simulink model "SigmaDelta"  (R2021b)
settings: Solver=VariableStepAuto  StartTime=0.0  StopTime=1  RelTol=1e-3
PreLoadFcn:
  | load DecFir.mat
undefined symbols (not defined in the file or in its folder): designMultirateFIR
libraries: dspmlti4 x6
settings Model: Creator=Utente  LastModifiedBy=Utente

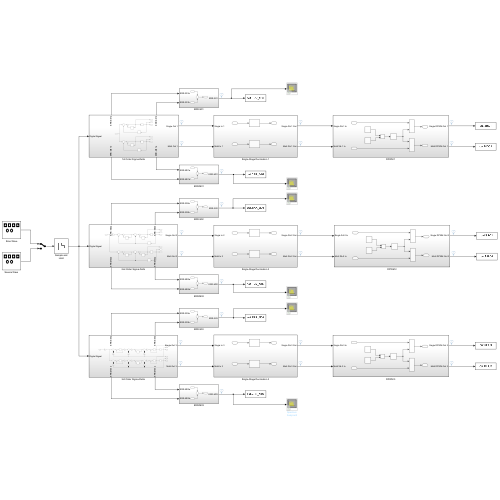
[thumbnail: Simulink's stored preview of the top-level diagram]
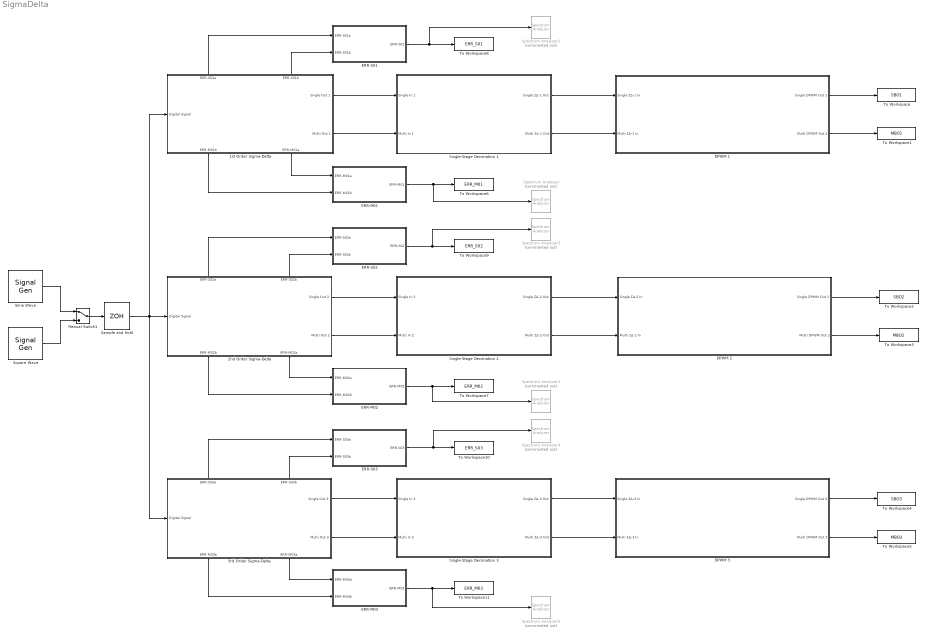
== system SigmaDelta ==
  "1st Order Sigma-Delta " : Subsystem
      settings: PortSchema="{\"entries\":[{\"content\":{\"sides\":[{\"content\":{\"connectorIds\":[\"In1\"]},\"type\":\"ConnectorPlacement.EquallySpacedRectSide\",\"uuid\":\"386a8987-fa85-4bfc-abbe-97ad6325c10a\"},{\"content\":{\"connectorIds\":[\"Out1\",\"Out2\"],\"side\":\"RIGHT\"},\"type\":\"ConnectorPlacement.EquallySpacedRectSide\",\"uuid\":\"605e7def-dc36-4f80-8847-9394a6da716c\"},{\"content\":{\"connectorIds\":[\"Out5\",\"Out6\"],\"side\":\"TOP\"},\"type\":\"ConnectorPlacement.EquallySpacedRectSide\",\"uuid\":\"bb7b67fd-46b8-47e1-a371-5b31483f4377\"},{\"content\":{\"connectorIds\":[\"Out3\",\"Out4\"],\"side\":\"BOTTOM\"},\"type\":\"ConnectorPlacement.EquallySpacedRectSide\",\"uuid\":\"407ca7d6-6743-42b4-90a6-330882115c21\"}]},\"type\":\"ConnectorPlacement.EquallySpacedConnector\",\"uuid\":\"38d6658d-cd74-4f08-86e0-cb3a607ff030\"}],\"packageUris\":[\"http://schema.mathworks.com/mf0/Connector/R2020b\"],\"version\":\"1.0\"}"
  2nd Order Sigma-Delta : Subsystem
      settings: PortSchema="{\"entries\":[{\"content\":{\"sides\":[{\"content\":{\"connectorIds\":[\"In1\"]},\"type\":\"ConnectorPlacement.EquallySpacedRectSide\",\"uuid\":\"386a8987-fa85-4bfc-abbe-97ad6325c10a\"},{\"content\":{\"connectorIds\":[\"Out1\",\"Out2\"],\"side\":\"RIGHT\"},\"type\":\"ConnectorPlacement.EquallySpacedRectSide\",\"uuid\":\"605e7def-dc36-4f80-8847-9394a6da716c\"},{\"content\":{\"connectorIds\":[\"Out5\",\"Out6\"],\"side\":\"TOP\"},\"type\":\"ConnectorPlacement.EquallySpacedRectSide\",\"uuid\":\"bb7b67fd-46b8-47e1-a371-5b31483f4377\"},{\"content\":{\"connectorIds\":[\"Out3\",\"Out4\"],\"side\":\"BOTTOM\"},\"type\":\"ConnectorPlacement.EquallySpacedRectSide\",\"uuid\":\"9f9d581d-12dd-4703-9574-97e4d852a146\"}]},\"type\":\"ConnectorPlacement.EquallySpacedConnector\",\"uuid\":\"38d6658d-cd74-4f08-86e0-cb3a607ff030\"}],\"packageUris\":[\"http://schema.mathworks.com/mf0/Connector/R2020b\"],\"version\":\"1.0\"}"
  3rd Order Sigma-Delta : Subsystem
      settings: PortSchema="{\"entries\":[{\"content\":{\"sides\":[{\"content\":{\"connectorIds\":[\"In1\"]},\"type\":\"ConnectorPlacement.EquallySpacedRectSide\",\"uuid\":\"358bd809-644a-47c9-aee6-c26862502fbd\"},{\"content\":{\"connectorIds\":[\"Out1\",\"Out2\"],\"side\":\"RIGHT\"},\"type\":\"ConnectorPlacement.EquallySpacedRectSide\",\"uuid\":\"63769fbe-dbed-44df-abee-7514b671db90\"},{\"content\":{\"connectorIds\":[\"Out5\",\"Out6\"],\"side\":\"TOP\"},\"type\":\"ConnectorPlacement.EquallySpacedRectSide\",\"uuid\":\"5696ef81-7309-4688-a911-424d4e0695b6\"},{\"content\":{\"connectorIds\":[\"Out3\",\"Out4\"],\"side\":\"BOTTOM\"},\"type\":\"ConnectorPlacement.EquallySpacedRectSide\",\"uuid\":\"575d4fed-9583-4a67-98b3-10e8b887a15e\"}]},\"type\":\"ConnectorPlacement.EquallySpacedConnector\",\"uuid\":\"3f568709-b940-42e7-9c29-4ecbd340a24d\"}],\"packageUris\":[\"http://schema.mathworks.com/mf0/Connector/R2020b\"],\"version\":\"1.0\"}"
  DPWM 1 : Subsystem
  DPWM 2 : Subsystem
  DPWM 3 : Subsystem
  ERR-M01 : Subsystem
  ERR-M02 : Subsystem
  ERR-M03 : Subsystem
  ERR-S01 : Subsystem
  ERR-S02 : Subsystem
  ERR-S03 : Subsystem
  Manual Switch1 : ManualSwitch
  Sample and Hold : ZeroOrderHold  SampleTime=1/(48e3*64)
  Siine Wave : SignalGenerator  Frequency=6283  Units=rad/sec
  Single-Stage Decimation 1 : Subsystem
  Single-Stage Decimation 2 : Subsystem
  Single-Stage Decimation 3 : Subsystem
  Spectrum Analyzer{,1..5} (6 alike) : SpectrumAnalyzer  Commented=on
  Square Wave : SignalGenerator  WaveForm=square  Frequency=6283  Units=rad/sec
  To Workspace : ToWorkspace  VariableName=SBO1  SaveFormat=Timeseries  SampleTime=-1
  To Workspace1 : ToWorkspace  VariableName=MBO1  SaveFormat=Timeseries  SampleTime=-1
  To Workspace10 : ToWorkspace  VariableName=ERR_S03  SaveFormat=Timeseries  SampleTime=-1
  To Workspace11 : ToWorkspace  VariableName=ERR_M03  SaveFormat=Timeseries  SampleTime=-1
  To Workspace2 : ToWorkspace  VariableName=SBO2  SaveFormat=Timeseries  SampleTime=-1
  To Workspace3 : ToWorkspace  VariableName=MBO2  SaveFormat=Timeseries  SampleTime=-1
  To Workspace4 : ToWorkspace  VariableName=SBO3  SaveFormat=Timeseries  SampleTime=-1
  To Workspace5 : ToWorkspace  VariableName=MBO3  SaveFormat=Timeseries  SampleTime=-1
  To Workspace6 : ToWorkspace  VariableName=ERR_M01  SaveFormat=Timeseries  SampleTime=-1
  To Workspace7 : ToWorkspace  VariableName=ERR_M02  SaveFormat=Timeseries  SampleTime=-1
  To Workspace8 : ToWorkspace  VariableName=ERR_S01  SaveFormat=Timeseries  SampleTime=-1
  To Workspace9 : ToWorkspace  VariableName=ERR_S02  SaveFormat=Timeseries  SampleTime=-1
  wires:
  Square Wave/1 -> Manual Switch1/2
  DPWM 1/2(Multi DPWM Out 1) -> To Workspace1/1
  DPWM 1/1(Single DPWM Out 1) -> To Workspace/1
  3rd Order Sigma-Delta/2(Multi Out 3) -> Single-Stage Decimation 3/2(Multi In 3)
  3rd Order Sigma-Delta/1(Single Out 3) -> Single-Stage Decimation 3/1(Single In 3)
  Single-Stage Decimation 3/2(Multi ΣΔ-3 Out) -> DPWM 3/2(Multi ΣΔ-3 In)
  Single-Stage Decimation 3/1(Single ΣΔ-3 Out) -> DPWM 3/1(Single ΣΔ-3 In)
  DPWM 3/1(Single DPWM Out 3) -> To Workspace4/1
  Single-Stage Decimation 1/1(Single ΣΔ-1 Out) -> DPWM 1/1(Single ΣΔ-1 In)
  "1st Order Sigma-Delta "/2(" Multi Out 1") -> Single-Stage Decimation 1/2(Multi In 1)
  "1st Order Sigma-Delta "/1(Single Out 1) -> Single-Stage Decimation 1/1(Single In 1)
  DPWM 2/2(Multi DPWM Out 2) -> To Workspace3/1
  Manual Switch1/1 -> Sample and Hold/1
  DPWM 2/1(Single DPWM Out 2) -> To Workspace2/1
  Single-Stage Decimation 1/2(Multi ΣΔ-1 Out) -> DPWM 1/2(Multi ΣΔ-1 In)
  2nd Order Sigma-Delta/1(Single Out 2) -> Single-Stage Decimation 2/1(Single In 2)
  DPWM 3/2(Multi DPWM Out 3) -> To Workspace5/1
  Sample and Hold/1 -> "1st Order Sigma-Delta "/1(Digital Signal), 3rd Order Sigma-Delta/1(Digital Signal), 2nd Order Sigma-Delta/1(Digital Signal)
  Siine Wave/1 -> Manual Switch1/1
  Single-Stage Decimation 2/2(Multi ΣΔ-2 Out) -> DPWM 2/2(Multi ΣΔ-2 In)
  Single-Stage Decimation 2/1(Single ΣΔ-2 Out) -> DPWM 2/1(Single ΣΔ-2 In)
  2nd Order Sigma-Delta/2(" Multi Out 2") -> Single-Stage Decimation 2/2(Multi In 2)
  ERR-M01/1(ERR-M01) -> Spectrum Analyzer/1, To Workspace6/1
  "1st Order Sigma-Delta "/4(ERR-M01a) -> ERR-M01/1(ERR-M01a)
  "1st Order Sigma-Delta "/3(ERR-M01b) -> ERR-M01/2(ERR-M01b)
  2nd Order Sigma-Delta/4(ERR-M02a) -> ERR-M02/1(ERR-M02a)
  2nd Order Sigma-Delta/3(ERR-M02b) -> ERR-M02/2(ERR-M02b)
  ERR-S01/1(ERR-S01) -> Spectrum Analyzer2/1, To Workspace8/1
  "1st Order Sigma-Delta "/6(ERR-S01b) -> ERR-S01/2(ERR-S01b)
  "1st Order Sigma-Delta "/5(ERR-S01a) -> ERR-S01/1(ERR-S01a)
  ERR-S02/1(ERR-S02) -> Spectrum Analyzer3/1, To Workspace9/1
  2nd Order Sigma-Delta/5(ERR-S02a) -> ERR-S02/1(ERR-S02a)
  2nd Order Sigma-Delta/6(ERR-S02b) -> ERR-S02/2(ERR-S02b)
  ERR-M02/1(ERR-M02) -> Spectrum Analyzer1/1, To Workspace7/1
  3rd Order Sigma-Delta/6(ERR-S03b) -> ERR-S03/2(ERR-S03b)
  ERR-S03/1(ERR-S03) -> Spectrum Analyzer4/1, To Workspace10/1
  3rd Order Sigma-Delta/5(ERR-S03a) -> ERR-S03/1(ERR-S03a)
  3rd Order Sigma-Delta/3(ERR-M03b) -> ERR-M03/2(ERR-M03b)
  ERR-M03/1(ERR-M03) -> Spectrum Analyzer5/1, To Workspace11/1
  3rd Order Sigma-Delta/4(ERR-M03a) -> ERR-M03/1(ERR-M03a)

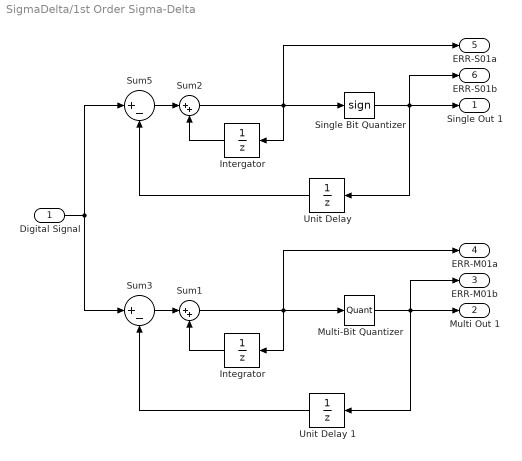
== system SigmaDelta/1st Order Sigma-Delta  ==
  Digital Signal : Inport
  Integrator : UnitDelay  SampleTime=-1  HasFrameUpgradeWarning=on
  Intergator : UnitDelay  SampleTime=-1  HasFrameUpgradeWarning=on
  Multi-Bit Quantizer : Quantizer  QuantizationInterval=0.15
  Single Bit Quantizer : Signum
  Sum1 : Sum  Inputs=|++
  Sum2 : Sum  Inputs=|++
  Sum3 : Sum  Inputs=|+-  AccumDataTypeStr=double  SampleTime=1/(48e3*64)
  Sum5 : Sum  Inputs=|+-  AccumDataTypeStr=double  SampleTime=1/(48e3*64)
  Unit Delay : UnitDelay  SampleTime=-1  HasFrameUpgradeWarning=on
  Unit Delay 1 : UnitDelay  SampleTime=-1  HasFrameUpgradeWarning=on
  Single Out 1 : Outport
  " Multi Out 1" : Outport  Port=2  OutDataTypeStr=double
  ERR-M01b : Outport  Port=3  OutDataTypeStr=double
  ERR-M01a : Outport  Port=4  OutDataTypeStr=double
  ERR-S01a : Outport  Port=5  OutDataTypeStr=double
  ERR-S01b : Outport  Port=6  OutDataTypeStr=double
  wires:
  Unit Delay/1 -> Sum5/2
  Intergator/1 -> Sum2/2
  Sum5/1 -> Sum2/1
  Unit Delay 1/1 -> Sum3/2
  Integrator/1 -> Sum1/2
  Digital Signal/1 -> Sum5/1, Sum3/1
  Sum3/1 -> Sum1/1
  Sum1/1 -> ERR-M01a/1, Multi-Bit Quantizer/1, Integrator/1
  Multi-Bit Quantizer/1 -> " Multi Out 1"/1, Unit Delay 1/1, ERR-M01b/1
  Sum2/1 -> ERR-S01a/1, Intergator/1, Single Bit Quantizer/1
  Single Bit Quantizer/1 -> ERR-S01b/1, Unit Delay/1, Single Out 1/1

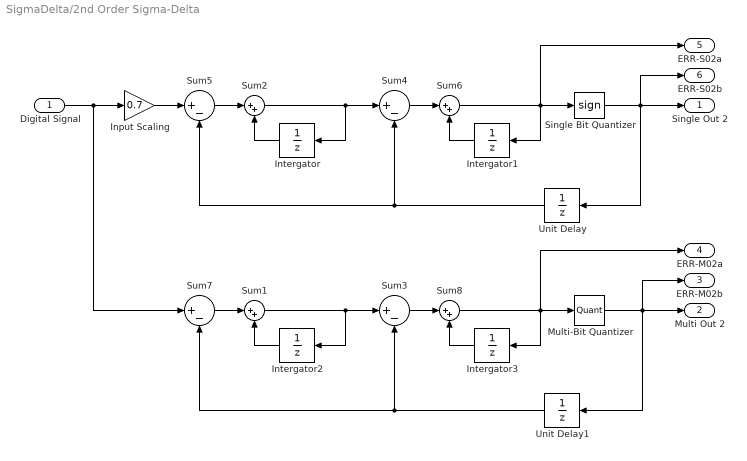
== system SigmaDelta/2nd Order Sigma-Delta ==
  Digital Signal : Inport
  Input Scaling : Gain  Gain=0.7  SampleTime=1/(48e3*64)
  Intergator{,1..3} (4 alike) : UnitDelay  SampleTime=-1  HasFrameUpgradeWarning=on
  Multi-Bit Quantizer : Quantizer  QuantizationInterval=0.15
  Single Bit Quantizer : Signum
  Sum{1..2,6,8} (4 alike) : Sum  Inputs=|++
  Sum{3..5,7} (4 alike) : Sum  Inputs=|+-  AccumDataTypeStr=double  SampleTime=1/(48e3*64)
  Unit Delay : UnitDelay  SampleTime=-1  HasFrameUpgradeWarning=on
  Unit Delay1 : UnitDelay  SampleTime=-1  HasFrameUpgradeWarning=on
  Single Out 2 : Outport
  " Multi Out 2" : Outport  Port=2  OutDataTypeStr=double
  ERR-M02b : Outport  Port=3  OutDataTypeStr=double
  ERR-M02a : Outport  Port=4  OutDataTypeStr=double
  ERR-S02a : Outport  Port=5  OutDataTypeStr=double
  ERR-S02b : Outport  Port=6  OutDataTypeStr=double
  wires:
  Sum2/1 -> Sum4/1, Intergator/1
  Unit Delay/1 -> Sum4/2, Sum5/2
  Intergator/1 -> Sum2/2
  Sum5/1 -> Sum2/1
  Input Scaling/1 -> Sum5/1
  Sum4/1 -> Sum6/1
  Intergator1/1 -> Sum6/2
  Sum3/1 -> Sum8/1
  Sum7/1 -> Sum1/1
  Intergator2/1 -> Sum1/2
  Sum1/1 -> Sum3/1, Intergator2/1
  Unit Delay1/1 -> Sum3/2, Sum7/2
  Digital Signal/1 -> Sum7/1, Input Scaling/1
  Intergator3/1 -> Sum8/2
  Sum8/1 -> ERR-M02a/1, Multi-Bit Quantizer/1, Intergator3/1
  Multi-Bit Quantizer/1 -> Unit Delay1/1, " Multi Out 2"/1, ERR-M02b/1
  Sum6/1 -> ERR-S02a/1, Single Bit Quantizer/1, Intergator1/1
  Single Bit Quantizer/1 -> Unit Delay/1, ERR-S02b/1, Single Out 2/1

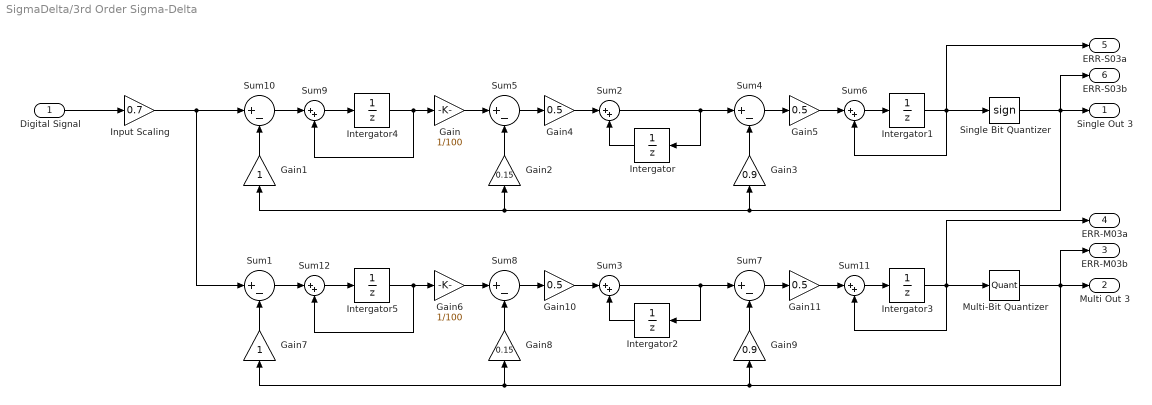
== system SigmaDelta/3rd Order Sigma-Delta ==
  Digital Signal : Inport
  Gain : Gain  Gain=1/100
  Gain1 : Gain
  Gain{4..5,10..11} (4 alike) : Gain  Gain=0.5
  Gain2 : Gain  Gain=0.15
  Gain3 : Gain  Gain=0.9
  Gain6 : Gain  Gain=1/100
  Gain7 : Gain
  Gain8 : Gain  Gain=0.15
  Gain9 : Gain  Gain=0.9
  Input Scaling : Gain  Gain=0.7  SampleTime=1/(48e3*64)
  Intergator{,1..5} (6 alike) : UnitDelay  SampleTime=-1  HasFrameUpgradeWarning=on
  Multi-Bit Quantizer : Quantizer  QuantizationInterval=0.15
  Single Bit Quantizer : Signum
  Sum{1,4..5,7..8,10} (6 alike) : Sum  Inputs=|+-  AccumDataTypeStr=double  SampleTime=1/(48e3*64)
  Sum{2..3,6,9,11..12} (6 alike) : Sum  Inputs=|++
  Single Out 3 : Outport
  Multi Out 3 : Outport  Port=2
  ERR-M03b : Outport  Port=3  OutDataTypeStr=double
  ERR-M03a : Outport  Port=4  OutDataTypeStr=double
  ERR-S03a : Outport  Port=5  OutDataTypeStr=double
  ERR-S03b : Outport  Port=6  OutDataTypeStr=double
  wires:
  Sum2/1 -> Sum4/1, Intergator/1
  Intergator/1 -> Sum2/2
  Sum5/1 -> Gain4/1
  Sum6/1 -> Intergator1/1
  Digital Signal/1 -> Input Scaling/1
  Sum10/1 -> Sum9/1
  Sum9/1 -> Intergator4/1
  Intergator4/1 -> Gain/1, Sum9/2
  Gain/1 -> Sum5/1
  Gain1/1 -> Sum10/2
  Gain2/1 -> Sum5/2
  Gain3/1 -> Sum4/2
  Gain4/1 -> Sum2/1
  Sum4/1 -> Gain5/1
  Gain5/1 -> Sum6/1
  Gain7/1 -> Sum1/2
  Intergator5/1 -> Gain6/1, Sum12/2
  Sum12/1 -> Intergator5/1
  Sum1/1 -> Sum12/1
  Gain9/1 -> Sum7/2
  Sum7/1 -> Gain11/1
  Sum11/1 -> Intergator3/1
  Gain10/1 -> Sum3/1
  Sum8/1 -> Gain10/1
  Intergator2/1 -> Sum3/2
  Gain6/1 -> Sum8/1
  Input Scaling/1 -> Sum1/1, Sum10/1
  Gain11/1 -> Sum11/1
  Gain8/1 -> Sum8/2
  Sum3/1 -> Sum7/1, Intergator2/1
  Intergator3/1 -> ERR-M03a/1, Multi-Bit Quantizer/1, Sum11/2
  Multi-Bit Quantizer/1 -> ERR-M03b/1, Gain9/1, Gain7/1, Gain8/1, Multi Out 3/1
  Single Bit Quantizer/1 -> ERR-S03b/1, Gain3/1, Gain1/1, Gain2/1, Single Out 3/1
  Intergator1/1 -> ERR-S03a/1, Single Bit Quantizer/1, Sum6/2

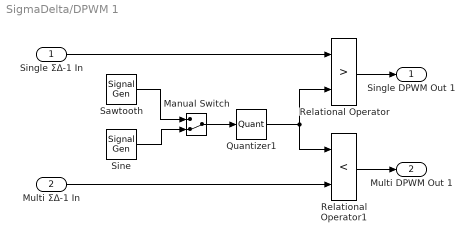
== system SigmaDelta/DPWM 1 ==
  Single ΣΔ-1 In : Inport
  Multi ΣΔ-1 In : Inport  Port=2
  Manual Switch : ManualSwitch  CurrentSetting=0
  Quantizer1 : Quantizer  QuantizationInterval=0.15
  Relational Operator : RelationalOperator  Operator=>  OutDataTypeStr=boolean  RndMeth=Simplest
  Relational Operator1 : RelationalOperator  Operator=<  OutDataTypeStr=boolean  RndMeth=Simplest
  Sawtooth : SignalGenerator  WaveForm=sawtooth  Frequency=1000  Units=rad/sec
  "Sine " : SignalGenerator  Frequency=1000  Units=rad/sec
  Single DPWM Out 1 : Outport
  Multi DPWM Out 1 : Outport  Port=2
  wires:
  Sawtooth/1 -> Manual Switch/1
  "Sine "/1 -> Manual Switch/2
  Manual Switch/1 -> Quantizer1/1
  Single ΣΔ-1 In/1 -> Relational Operator/1
  Quantizer1/1 -> Relational Operator/2, Relational Operator1/1
  Relational Operator/1 -> Single DPWM Out 1/1
  Relational Operator1/1 -> Multi DPWM Out 1/1
  Multi ΣΔ-1 In/1 -> Relational Operator1/2

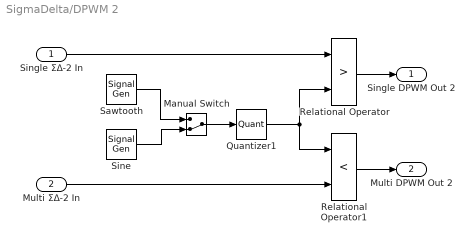
== system SigmaDelta/DPWM 2 ==
  Single ΣΔ-2 In : Inport
  Multi ΣΔ-2 In : Inport  Port=2
  Manual Switch : ManualSwitch  CurrentSetting=0
  Quantizer1 : Quantizer  QuantizationInterval=0.15
  Relational Operator : RelationalOperator  Operator=>  OutDataTypeStr=boolean  RndMeth=Simplest
  Relational Operator1 : RelationalOperator  Operator=<  OutDataTypeStr=boolean  RndMeth=Simplest
  Sawtooth : SignalGenerator  WaveForm=sawtooth  Frequency=1000  Units=rad/sec
  "Sine " : SignalGenerator  Frequency=1000  Units=rad/sec
  Single DPWM Out 2 : Outport
  Multi DPWM Out 2 : Outport  Port=2
  wires:
  Sawtooth/1 -> Manual Switch/1
  "Sine "/1 -> Manual Switch/2
  Manual Switch/1 -> Quantizer1/1
  Single ΣΔ-2 In/1 -> Relational Operator/1
  Quantizer1/1 -> Relational Operator/2, Relational Operator1/1
  Relational Operator/1 -> Single DPWM Out 2/1
  Relational Operator1/1 -> Multi DPWM Out 2/1
  Multi ΣΔ-2 In/1 -> Relational Operator1/2

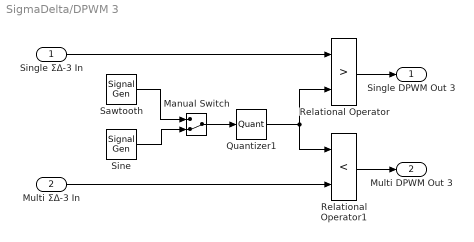
== system SigmaDelta/DPWM 3 ==
  Single ΣΔ-3 In : Inport
  Multi ΣΔ-3 In : Inport  Port=2
  Manual Switch : ManualSwitch  CurrentSetting=0
  Quantizer1 : Quantizer  QuantizationInterval=0.15
  Relational Operator : RelationalOperator  Operator=>  OutDataTypeStr=boolean  RndMeth=Simplest
  Relational Operator1 : RelationalOperator  Operator=<  OutDataTypeStr=boolean  RndMeth=Simplest
  Sawtooth : SignalGenerator  WaveForm=sawtooth  Frequency=1000  Units=rad/sec
  "Sine " : SignalGenerator  Frequency=1000  Units=rad/sec
  Single DPWM Out 3 : Outport
  Multi DPWM Out 3 : Outport  Port=2
  wires:
  Sawtooth/1 -> Manual Switch/1
  "Sine "/1 -> Manual Switch/2
  Manual Switch/1 -> Quantizer1/1
  Single ΣΔ-3 In/1 -> Relational Operator/1
  Quantizer1/1 -> Relational Operator/2, Relational Operator1/1
  Relational Operator/1 -> Single DPWM Out 3/1
  Relational Operator1/1 -> Multi DPWM Out 3/1
  Multi ΣΔ-3 In/1 -> Relational Operator1/2

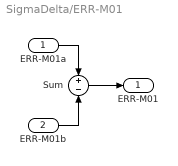
== system SigmaDelta/ERR-M01 ==
  ERR-M01a : Inport
  ERR-M01b : Inport  Port=2
  Sum : Sum  Inputs=+|-
  ERR-M01 : Outport
  wires:
  ERR-M01a/1 -> Sum/1
  ERR-M01b/1 -> Sum/2
  Sum/1 -> ERR-M01/1

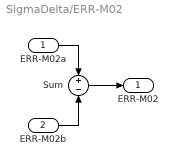
== system SigmaDelta/ERR-M02 ==
  ERR-M02a : Inport
  ERR-M02b : Inport  Port=2
  Sum : Sum  Inputs=+|-
  ERR-M02 : Outport
  wires:
  ERR-M02a/1 -> Sum/1
  ERR-M02b/1 -> Sum/2
  Sum/1 -> ERR-M02/1

== system SigmaDelta/ERR-M03 ==
  ERR-M03a : Inport
  ERR-M03b : Inport  Port=2
  Sum : Sum  Inputs=+|-
  ERR-M03 : Outport
  wires:
  ERR-M03a/1 -> Sum/1
  ERR-M03b/1 -> Sum/2
  Sum/1 -> ERR-M03/1

== system SigmaDelta/ERR-S01 ==
  ERR-S01a : Inport
  ERR-S01b : Inport  Port=2
  Sum : Sum  Inputs=+|-
  ERR-S01 : Outport
  wires:
  ERR-S01a/1 -> Sum/1
  ERR-S01b/1 -> Sum/2
  Sum/1 -> ERR-S01/1

== system SigmaDelta/ERR-S02 ==
  ERR-S02a : Inport
  ERR-S02b : Inport  Port=2
  Sum : Sum  Inputs=+|-
  ERR-S02 : Outport
  wires:
  ERR-S02a/1 -> Sum/1
  ERR-S02b/1 -> Sum/2
  Sum/1 -> ERR-S02/1

== system SigmaDelta/ERR-S03 ==
  ERR-S03a : Inport
  ERR-S03b : Inport  Port=2
  Sum : Sum  Inputs=+|-
  ERR-S03 : Outport
  wires:
  ERR-S03a/1 -> Sum/1
  ERR-S03b/1 -> Sum/2
  Sum/1 -> ERR-S03/1

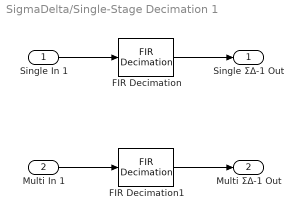
== system SigmaDelta/Single-Stage Decimation 1 ==
  Single In 1 : Inport
  Multi In 1 : Inport  Port=2
  FIR Decimation : dspmlti4/FIR Decimation  FilterSource=Filter object  h=designMultirateFIR(1,2)  D=2  filtStruct=Direct form  FilterObject=h  InputProcessing=Columns as channels (frame based)  framing=Allow multirate processing  inputOffset=0  outputBufInitCond=0  roundingMode=Floor  overflowMode=off  firstCoeffDataTypeStr=Inherit: Same word length as input  firstCoeffMin=[]  firstCoeffMax=[]  firstCoeffLastDataTypeStr=Inherit: Same word length as input  outputDataTypeStr=Inherit: Same as accumulator  outputMin=[]  outputMax=[]  outputLastDataTypeStr=Inherit: Same as accumulator
  FIR Decimation1 : dspmlti4/FIR Decimation  FilterSource=Filter object  h=designMultirateFIR(1,2)  D=2  filtStruct=Direct form  FilterObject=h  InputProcessing=Columns as channels (frame based)  framing=Allow multirate processing  inputOffset=0  outputBufInitCond=0  roundingMode=Floor  overflowMode=off  firstCoeffDataTypeStr=Inherit: Same word length as input  firstCoeffMin=[]  firstCoeffMax=[]  firstCoeffLastDataTypeStr=Inherit: Same word length as input  outputDataTypeStr=Inherit: Same as accumulator  outputMin=[]  outputMax=[]  outputLastDataTypeStr=Inherit: Same as accumulator
  Single ΣΔ-1 Out : Outport
  Multi ΣΔ-1 Out : Outport  Port=2
  wires:
  Single In 1/1 -> FIR Decimation/1
  FIR Decimation1/1 -> Multi ΣΔ-1 Out/1
  Multi In 1/1 -> FIR Decimation1/1
  FIR Decimation/1 -> Single ΣΔ-1 Out/1

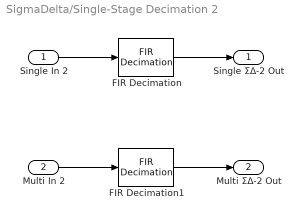
== system SigmaDelta/Single-Stage Decimation 2 ==
  Single In 2 : Inport
  Multi In 2 : Inport  Port=2
  FIR Decimation : dspmlti4/FIR Decimation  FilterSource=Filter object  h=designMultirateFIR(1,2)  D=2  filtStruct=Direct form  FilterObject=h  InputProcessing=Columns as channels (frame based)  framing=Allow multirate processing  inputOffset=0  outputBufInitCond=0  roundingMode=Floor  overflowMode=off  firstCoeffDataTypeStr=Inherit: Same word length as input  firstCoeffMin=[]  firstCoeffMax=[]  firstCoeffLastDataTypeStr=Inherit: Same word length as input  outputDataTypeStr=Inherit: Same as accumulator  outputMin=[]  outputMax=[]  outputLastDataTypeStr=Inherit: Same as accumulator
  FIR Decimation1 : dspmlti4/FIR Decimation  FilterSource=Filter object  h=designMultirateFIR(1,2)  D=2  filtStruct=Direct form  FilterObject=h  InputProcessing=Columns as channels (frame based)  framing=Allow multirate processing  inputOffset=0  outputBufInitCond=0  roundingMode=Floor  overflowMode=off  firstCoeffDataTypeStr=Inherit: Same word length as input  firstCoeffMin=[]  firstCoeffMax=[]  firstCoeffLastDataTypeStr=Inherit: Same word length as input  outputDataTypeStr=Inherit: Same as accumulator  outputMin=[]  outputMax=[]  outputLastDataTypeStr=Inherit: Same as accumulator
  Single ΣΔ-2 Out : Outport
  Multi ΣΔ-2 Out : Outport  Port=2
  wires:
  FIR Decimation1/1 -> Multi ΣΔ-2 Out/1
  Multi In 2/1 -> FIR Decimation1/1
  FIR Decimation/1 -> Single ΣΔ-2 Out/1
  Single In 2/1 -> FIR Decimation/1

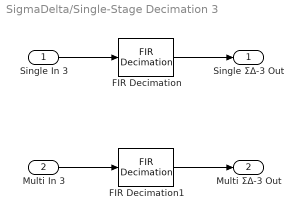
== system SigmaDelta/Single-Stage Decimation 3 ==
  Single In 3 : Inport
  Multi In 3 : Inport  Port=2
  FIR Decimation : dspmlti4/FIR Decimation  FilterSource=Filter object  h=designMultirateFIR(1,2)  D=2  filtStruct=Direct form  FilterObject=h  InputProcessing=Columns as channels (frame based)  framing=Allow multirate processing  inputOffset=0  outputBufInitCond=0  roundingMode=Floor  overflowMode=off  firstCoeffDataTypeStr=Inherit: Same word length as input  firstCoeffMin=[]  firstCoeffMax=[]  firstCoeffLastDataTypeStr=Inherit: Same word length as input  outputDataTypeStr=Inherit: Same as accumulator  outputMin=[]  outputMax=[]  outputLastDataTypeStr=Inherit: Same as accumulator
  FIR Decimation1 : dspmlti4/FIR Decimation  FilterSource=Filter object  h=designMultirateFIR(1,2)  D=2  filtStruct=Direct form  FilterObject=h  InputProcessing=Columns as channels (frame based)  framing=Allow multirate processing  inputOffset=0  outputBufInitCond=0  roundingMode=Floor  overflowMode=off  firstCoeffDataTypeStr=Inherit: Same word length as input  firstCoeffMin=[]  firstCoeffMax=[]  firstCoeffLastDataTypeStr=Inherit: Same word length as input  outputDataTypeStr=Inherit: Same as accumulator  outputMin=[]  outputMax=[]  outputLastDataTypeStr=Inherit: Same as accumulator
  Single ΣΔ-3 Out : Outport
  Multi ΣΔ-3 Out : Outport  Port=2
  wires:
  FIR Decimation1/1 -> Multi ΣΔ-3 Out/1
  Multi In 3/1 -> FIR Decimation1/1
  FIR Decimation/1 -> Single ΣΔ-3 Out/1
  Single In 3/1 -> FIR Decimation/1
